simulink model "sampleModel1634"  (R2023a)
settings: Solver=VariableStepAuto  StartTime=0.0  StopTime=10.0  RelTol=1e-3
libraries: simulink x3, hdlsllib x2
settings Model: Creator=user1  LastModifiedBy=user1

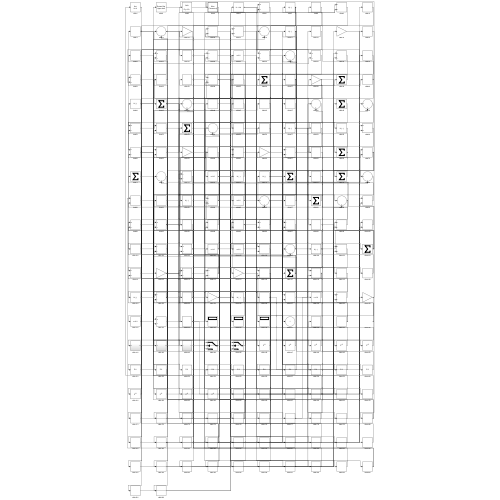
[thumbnail: Simulink's stored preview of the top-level diagram]
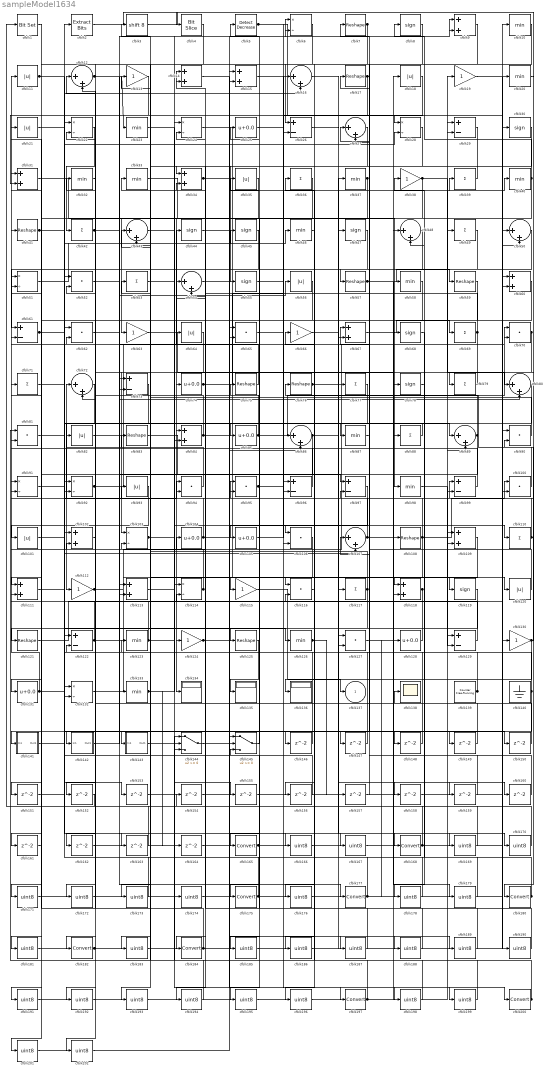
== system sampleModel1634 ==
  cfblk1 : simulink/Logic and Bit Operations/Bit Set  iBit=0
      settings: LibrarySourceBlock=|
      | hdlsllib/Logic and Bit
      | Operations/Bit Set
  cfblk{10,20,23,32..33,37,40,46,58,87,98,123,126,133} (14 alike) : MinMax
  cfblk{52,62,65,70,81,90,94..95,100,106,116,127} (12 alike) : DotProduct  OutDataTypeStr=Inherit: Inherit via internal rule
  cfblk{11,18,21,35,56,64,82,93,101,120} (10 alike) : Abs  SaturateOnIntegerOverflow=off
  cfblk{9,14..15,31,34,60,67,84,102,109,111,113,118} (13 alike) : Sum
  cfblk{6,22,24,28,51,91..92,103,114,132} (10 alike) : Product  Inputs=*/  RndMeth=Zero  SaturateOnIntegerOverflow=on
  cfblk{25,74,85,104..105,128,131} (7 alike) : Bias  Bias=0.0  SaturateOnIntegerOverflow=off
  cfblk{12,16,27,43,48,50,54,72,80,86,89,107} (12 alike) : Sum  Inputs=|++
  cfblk{7,17,41,57,59,75..76,83,108,121,125} (11 alike) : Reshape
  cfblk{36,39,42,49,53,69,71,77,79,88,110,117} (12 alike) : Sum  Inputs=+
  cfblk{13,19,38,63,66,112,115,124,130} (9 alike) : Gain
  cfblk{8,30,44..45,47,55,68,78,119} (9 alike) : Signum
  cfblk{26,29,61,73,96..97,99,122,129} (9 alike) : Sum  Inputs=+-
  cfblk134 : Display
  cfblk135 : Display
  cfblk136 : Display
  cfblk138 : Scope
  cfblk139 : hdlsllib/Sources/Counter Free-Running  NumBits=16  tsamp=-1
  cfblk140 : Ground
  cfblk141 : Subsystem
      settings: LibrarySourceBlock=|
      | hdlsllib/Ports &
      | Subsystems/Subsystem
  cfblk142 : Subsystem
      settings: LibrarySourceBlock=|
      | hdlsllib/Ports &
      | Subsystems/Subsystem
  cfblk143 : Subsystem
      settings: LibrarySourceBlock=|
      | hdlsllib/Ports &
      | Subsystems/Subsystem
  cfblk144 : Switch  SaturateOnIntegerOverflow=off  InputSameDT=off
  cfblk145 : Switch  SaturateOnIntegerOverflow=off  InputSameDT=off
  cfblk{146..164} (19 alike) : Delay  SampleTime=1
  cfblk{165,168,175,177,180,182,184,197,200} (9 alike) : DataTypeConversion  SaturateOnIntegerOverflow=off  RndMeth=Floor
  cfblk{166..167,169..174,176,178..179,181,183,185..196,198..199,201..202} (29 alike) : DataTypeConversion  OutDataTypeStr=uint8  SaturateOnIntegerOverflow=off  RndMeth=Floor
  cfblk2 : simulink/Logic and Bit Operations/Extract Bits  bitsToExtract=Upper half  numBits=8  bitIdxRange=[0 7]  outScalingMode=Preserve fixed-point scaling
      settings: LibrarySourceBlock=|
      | hdlsllib/Logic and Bit
      | Operations/Extract Bits
  cfblk3 : ArithShift  BitShiftNumber=8
  cfblk4 : hdlsllib/Logic and Bit Operations/Bit Slice  lidx=7  ridx=0
  cfblk5 : simulink/Logic and Bit Operations/Detect Decrease  vinit=0.0  OutDataTypeStr=boolean
      settings: LibrarySourceBlock=|
      | hdlsllib/Logic and Bit
      | Operations/Detect
      | Decrease
  cfblk137 : Outport  VectorParamsAs1DForOutWhenUnconnected=off
  wires:
  cfblk34/1 -> cfblk120/1, cfblk189/1
  cfblk45/1 -> cfblk134/1
  cfblk126/1 -> cfblk157/1, cfblk176/1
  cfblk133/1 -> cfblk114/1, cfblk164/1
  cfblk22/1 -> cfblk42/1
  cfblk27/1 -> cfblk55/1
  cfblk131/1 -> cfblk11/1, cfblk28/2
  cfblk60/1 -> cfblk184/1
  cfblk31/1 -> cfblk98/1
  cfblk114/1 -> cfblk41/1, cfblk51/2
  cfblk38/1 -> cfblk63/1, cfblk80/1, cfblk115/1
  cfblk7/1 -> cfblk26/1, cfblk106/1, cfblk186/1
  cfblk32/1 -> cfblk12/2
  cfblk130/1 -> cfblk99/1, cfblk196/1
  cfblk48/1 -> cfblk61/1
  cfblk100/1 -> cfblk76/1
  cfblk41/1 -> cfblk89/1, cfblk16/2
  cfblk64/1 -> cfblk103/1
  cfblk116/1 -> cfblk136/1
  cfblk68/1 -> cfblk118/1
  cfblk52/1 -> cfblk177/1
  cfblk3/1 -> cfblk79/1
  cfblk40/1 -> cfblk8/1, cfblk162/1
  cfblk51/1 -> cfblk45/1
  cfblk132/1 -> cfblk70/1
  cfblk80/1 -> cfblk112/1
  cfblk13/1 -> cfblk101/1
  cfblk110/1 -> cfblk72/1, cfblk75/1, cfblk90/2
  cfblk35/1 -> cfblk74/1
  cfblk113/1 -> cfblk24/1
  cfblk1/1 -> cfblk121/1
  cfblk121/1 -> cfblk37/1
  cfblk140/1 -> cfblk103/2, cfblk95/1, cfblk191/1
  cfblk39/1 -> cfblk34/1
  cfblk87/1 -> cfblk27/1
  cfblk20/1 -> cfblk180/1
  cfblk61/1 -> cfblk132/1, cfblk107/2
  cfblk67/1 -> cfblk69/1
  cfblk36/1 -> cfblk175/1
  cfblk72/1 -> cfblk92/2
  cfblk107/1 -> cfblk31/1, cfblk119/1
  cfblk8/1 -> cfblk87/1
  cfblk4/1 -> cfblk142/1(In1)
  cfblk57/1 -> cfblk59/1, cfblk179/1
  cfblk12/1 -> cfblk23/1, cfblk96/2
  cfblk24/1 -> cfblk127/1
  cfblk109/1 -> cfblk165/1
  cfblk141/1(Out1) -> cfblk94/1
  cfblk76/1 -> cfblk117/1, cfblk39/1
  cfblk127/1 -> cfblk48/1
  cfblk75/1 -> cfblk21/1
  cfblk91/1 -> cfblk46/1
  cfblk82/1 -> cfblk50/1
  cfblk103/1 -> cfblk13/1, cfblk6/2
  cfblk88/1 -> cfblk85/1
  cfblk2/1 -> cfblk4/1
  cfblk30/1 -> cfblk143/1(In1)
  cfblk23/1 -> cfblk110/1
  cfblk65/1 -> cfblk200/1
  cfblk56/1 -> cfblk111/1
  cfblk90/1 -> cfblk53/1
  cfblk112/1 -> cfblk116/1, cfblk64/1, cfblk166/1
  cfblk142/1(Out1) -> cfblk56/1
  cfblk28/1 -> cfblk57/1
  cfblk115/1 -> cfblk137/1
  cfblk59/1 -> cfblk68/1
  cfblk37/1 -> cfblk51/1, cfblk73/2
  cfblk47/1 -> cfblk124/1
  cfblk120/1 -> cfblk7/1
  cfblk98/1 -> cfblk129/2
  cfblk125/1 -> cfblk135/1
  cfblk97/1 -> cfblk105/1
  cfblk69/1 -> cfblk33/1, cfblk172/1
  cfblk43/1 -> cfblk197/1
  cfblk128/1 -> cfblk125/1
  cfblk5/1 -> cfblk50/2, cfblk28/1
  cfblk94/1 -> cfblk82/1
  cfblk104/1 -> cfblk94/2, cfblk86/2
  cfblk86/1 -> cfblk131/1, cfblk158/1, cfblk159/1
  cfblk92/1 -> cfblk44/1, cfblk80/2
  cfblk101/1 -> cfblk2/1
  cfblk74/1 -> cfblk26/2, cfblk106/2
  cfblk21/1 -> cfblk102/1
  cfblk58/1 -> cfblk141/1(In1)
  cfblk129/1 -> cfblk22/2
  cfblk17/1 -> cfblk27/2, cfblk31/2, cfblk67/2
  cfblk84/1 -> cfblk32/1, cfblk146/1
  cfblk123/1 -> cfblk71/1, cfblk167/1
  cfblk105/1 -> cfblk16/1
  cfblk25/1 -> cfblk96/1
  cfblk99/1 -> cfblk38/1
  cfblk11/1 -> cfblk126/1, cfblk144/3
  cfblk77/1 -> cfblk182/1
  cfblk118/1 -> cfblk111/2, cfblk144/2
  cfblk79/1 -> cfblk78/1
  cfblk95/1 -> cfblk169/1, cfblk195/1
  cfblk124/1 -> cfblk40/1, cfblk199/1
  cfblk85/1 -> cfblk70/2, cfblk14/1
  cfblk62/1 -> cfblk6/1
  cfblk144/1 -> cfblk9/1
  cfblk96/1 -> cfblk5/1
  cfblk108/1 -> cfblk100/1, cfblk25/1, cfblk185/1
  cfblk139/1 -> cfblk17/1, cfblk102/2
  cfblk63/1 -> cfblk108/1
  cfblk145/1 -> cfblk35/1
  cfblk44/1 -> cfblk9/2
  cfblk66/1 -> cfblk168/1
  cfblk117/1 -> cfblk93/1, cfblk83/1, cfblk161/1
  cfblk89/1 -> cfblk81/2, cfblk95/2, cfblk67/1
  cfblk70/1 -> cfblk84/1, cfblk84/2
  cfblk73/1 -> cfblk113/2
  cfblk83/1 -> cfblk97/1
  cfblk122/1 -> cfblk30/1, cfblk91/1
  cfblk42/1 -> cfblk133/1, cfblk88/1
  cfblk33/1 -> cfblk86/1
  cfblk146/1 -> cfblk113/1
  cfblk9/1 -> cfblk147/1
  cfblk147/1 -> cfblk92/1
  cfblk26/1 -> cfblk148/1
  cfblk148/1 -> cfblk24/2
  cfblk111/1 -> cfblk149/1
  cfblk149/1 -> cfblk73/1
  cfblk14/1 -> cfblk150/1
  cfblk150/1 -> cfblk12/1
  cfblk6/1 -> cfblk151/1
  cfblk151/1 -> cfblk132/2
  cfblk102/1 -> cfblk152/1
  cfblk152/1 -> cfblk1/1
  cfblk81/1 -> cfblk153/1
  cfblk153/1 -> cfblk89/2
  cfblk154/1 -> cfblk114/2
  cfblk143/1(Out1) -> cfblk155/1
  cfblk155/1 -> cfblk99/2
  cfblk46/1 -> cfblk156/1
  cfblk156/1 -> cfblk122/1
  cfblk157/1 -> cfblk107/1
  cfblk158/1 -> cfblk100/2
  cfblk159/1 -> cfblk48/2
  cfblk16/1 -> cfblk160/1
  cfblk160/1 -> cfblk97/2
  cfblk161/1 -> cfblk61/2
  cfblk162/1 -> cfblk129/1
  cfblk71/1 -> cfblk163/1
  cfblk163/1 -> cfblk22/1
  cfblk164/1 -> cfblk127/2
  cfblk165/1 -> cfblk90/1, cfblk58/1
  cfblk166/1 -> cfblk109/1
  cfblk167/1 -> cfblk109/2
  cfblk168/1 -> cfblk34/2, cfblk130/1
  cfblk169/1 -> cfblk66/1
  cfblk15/1 -> cfblk170/1
  cfblk170/1 -> cfblk62/1
  cfblk18/1 -> cfblk171/1
  cfblk171/1 -> cfblk15/1
  cfblk172/1 -> cfblk15/2
  cfblk10/1 -> cfblk173/1
  cfblk173/1 -> cfblk62/2
  cfblk53/1 -> cfblk174/1
  cfblk174/1 -> cfblk10/1
  cfblk175/1 -> cfblk154/1, cfblk122/2
  cfblk176/1 -> cfblk36/1
  cfblk177/1 -> cfblk14/2, cfblk128/1
  cfblk78/1 -> cfblk178/1
  cfblk178/1 -> cfblk52/1
  cfblk179/1 -> cfblk52/2
  cfblk180/1 -> cfblk138/1, cfblk104/1
  cfblk93/1 -> cfblk181/1
  cfblk181/1 -> cfblk20/1
  cfblk182/1 -> cfblk118/2, cfblk202/1
  cfblk106/1 -> cfblk183/1
  cfblk183/1 -> cfblk77/1
  cfblk184/1 -> cfblk123/1, cfblk91/2, cfblk72/2, cfblk47/1, cfblk198/1
  cfblk185/1 -> cfblk60/1
  cfblk186/1 -> cfblk60/2
  cfblk54/1 -> cfblk187/1
  cfblk187/1 -> cfblk145/3
  cfblk55/1 -> cfblk188/1
  cfblk188/1 -> cfblk54/1
  cfblk189/1 -> cfblk54/2
  cfblk19/1 -> cfblk190/1
  cfblk190/1 -> cfblk145/1
  cfblk191/1 -> cfblk19/1
  cfblk49/1 -> cfblk192/1
  cfblk192/1 -> cfblk145/2
  cfblk50/1 -> cfblk193/1
  cfblk193/1 -> cfblk49/1
  cfblk29/1 -> cfblk194/1
  cfblk194/1 -> cfblk81/1
  cfblk195/1 -> cfblk29/1
  cfblk196/1 -> cfblk29/2
  cfblk197/1 -> cfblk18/1, cfblk116/2
  cfblk198/1 -> cfblk43/1
  cfblk199/1 -> cfblk43/2
  cfblk200/1 -> cfblk144/1, cfblk3/1
  cfblk119/1 -> cfblk201/1
  cfblk201/1 -> cfblk65/1
  cfblk202/1 -> cfblk65/2

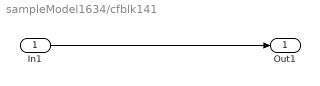
== system sampleModel1634/cfblk141 ==
  In1 : Inport
  Out1 : Outport
  wires:
  In1/1 -> Out1/1

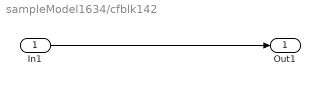
== system sampleModel1634/cfblk142 ==
  In1 : Inport
  Out1 : Outport
  wires:
  In1/1 -> Out1/1

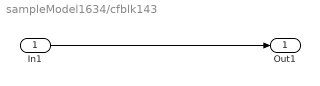
== system sampleModel1634/cfblk143 ==
  In1 : Inport
  Out1 : Outport
  wires:
  In1/1 -> Out1/1
